simulink model "aufgabe23ABC"  (R2014a)
settings: Solver=ode5  StartTime=0.0  StopTime=10.0  FixedStep=0.01  RelTol=1e-3
settings Model: Creator=s55812  LastModifiedBy=s55812

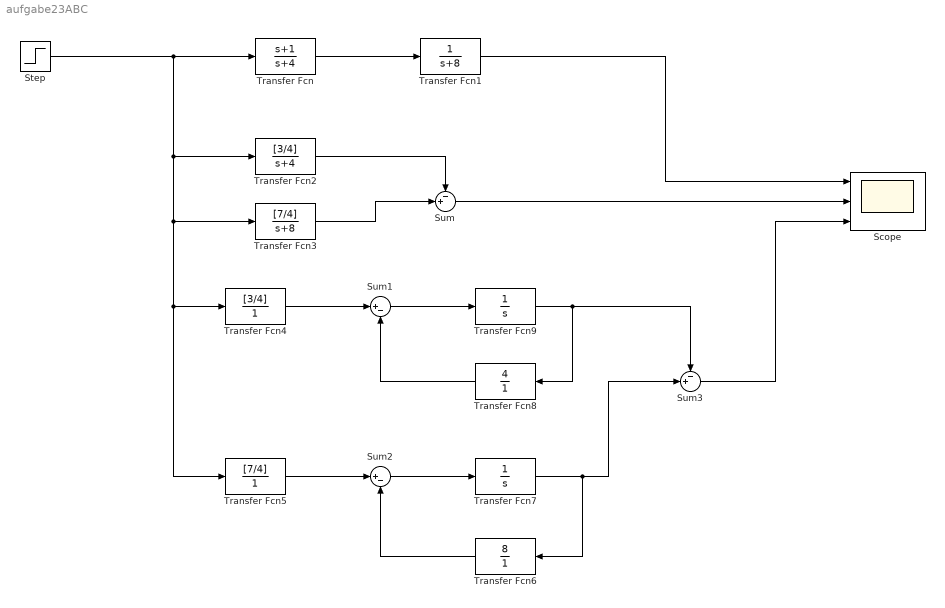
== system aufgabe23ABC ==
  Scope : Scope  NumInputPorts=3
      settings: YMin=-5~-5~-5  YMax=5~5~5
  Step : Step  SampleTime=0
  Sum : Sum  Inputs=-+|
  Sum1 : Sum  Inputs=|+-
  Sum2 : Sum  Inputs=|+-
  Sum3 : Sum  Inputs=-+|
  Transfer Fcn : TransferFcn  Numerator=[1 1]  Denominator=[1 4]
  Transfer Fcn1 : TransferFcn  Denominator=[1 8]
  Transfer Fcn2 : TransferFcn  Numerator=[3/4]  Denominator=[1 4]
  Transfer Fcn3 : TransferFcn  Numerator=[7/4]  Denominator=[1 8]
  Transfer Fcn4 : TransferFcn  Numerator=[3/4]  Denominator=[1]
  Transfer Fcn5 : TransferFcn  Numerator=[7/4]  Denominator=[1]
  Transfer Fcn6 : TransferFcn  Numerator=[8]  Denominator=[1]
  Transfer Fcn7 : TransferFcn  Denominator=[1 0]
  Transfer Fcn8 : TransferFcn  Numerator=[4]  Denominator=[1]
  Transfer Fcn9 : TransferFcn  Denominator=[1 0]
  wires:
  Step/1 -> Transfer Fcn5/1, Transfer Fcn4/1, Transfer Fcn3/1, Transfer Fcn2/1, Transfer Fcn/1
  Transfer Fcn/1 -> Transfer Fcn1/1
  Transfer Fcn1/1 -> Scope/1
  Transfer Fcn2/1 -> Sum/1
  Transfer Fcn3/1 -> Sum/2
  Sum/1 -> Scope/2
  Transfer Fcn4/1 -> Sum1/1
  Transfer Fcn5/1 -> Sum2/1
  Sum1/1 -> Transfer Fcn9/1
  Sum2/1 -> Transfer Fcn7/1
  Transfer Fcn7/1 -> Transfer Fcn6/1, Sum3/2
  Transfer Fcn9/1 -> Transfer Fcn8/1, Sum3/1
  Transfer Fcn8/1 -> Sum1/2
  Transfer Fcn6/1 -> Sum2/2
  Sum3/1 -> Scope/3
